simulink subsystem "StreetLaneSegment1x1_asSubsystem"  (R2021a)
settings: Solver=VariableStepAuto  StartTime=0.0  StopTime=10.0  RelTol=1e-3
settings Model: Creator=phill  LastModifiedBy=phill

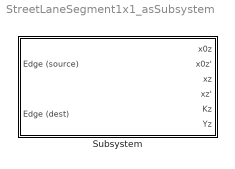
== system StreetLaneSegment1x1_asSubsystem ==
  Subsystem : Subsystem  mask{Kz=10, Tz=5}
      mask prompts: Kz "Kz (Capacity - How many cars fit into this cell)"; Tz "Tz (Nominal travel time for vehicles traveling unobstructed through the cell)"
      mask help:
      | This Block models a single Street-Lane capable of holding / transducing cars (or at least "car volume units") as a cell. This 1x1 version It is connected to a single source edge (over which it can receive cars from a preceeding cell) and a single destination edge (over which it can lose cars to the succeeding cell).  It has a capacity (how many volume-units of cars can be present on the segment at a given time) and a nominal travel time (how long cars would need to travel through it unobstructed). The outputs are:
      |
      | x0z  : how many cars (in car volume units) are "at the end of the cell" (and thus visible for the destination-edge  or the following cell).  The value can only rise if more cars flow in (mind the delay Tz!) than flow out - for instance if a traffic light blocks the exit.
      | x0z' : how many cars flow into (when positive sign) or out of (when negative) the cell
      | xz    : how many cars are in the cell in total (both the ones who just entered and have not reached the end yet, as well as the ones at the end)
      | xz'   : how many cars are flowing into- (positive sign) or out of (negative) the cell per time
      | yz    : the internal flow - how many cars pass into the "endpart" of a cell. It is delayed by Tz compared to the incoming flow y_incoming, so any cars that enter a cell will only "appear visible" at the end of it after that time Tz.
      mask Display:
      | disp('Street Lane Segment 1x1 \n\n');
      | disp(['Kz = ', get_param(gcb,'Kz'), ' | Tz = ', get_param(gcb, 'Tz')])

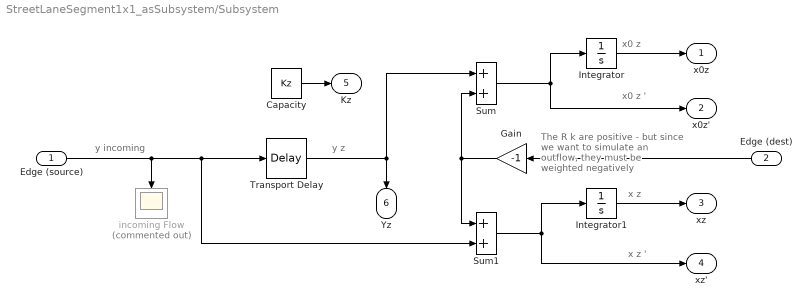
== system StreetLaneSegment1x1_asSubsystem/Subsystem ==
  note: y incoming
  note: x z '
  note: x z
  note: x0 z
  note: x0 z '
  note: y z
  note: The R k are positive - but since we
      | want to simulate an outflow, they
      | must be weighted negatively
  Edge (source) : Inport
  Edge (dest) : Inport  Port=2
  Capacity : Constant  Value=Kz
  Gain : Gain  Gain=-1
  Integrator : Integrator
  Integrator1 : Integrator
  Sum : Sum
  Sum1 : Sum
  Transport Delay : TransportDelay  DelayTime=Tz
  incoming Flow : Scope  Commented=on
  x0z : Outport
  x0z' : Outport  Port=2
  xz : Outport  Port=3
  xz' : Outport  Port=4
  Kz : Outport  Port=5
  Yz : Outport  Port=6
  wires:
  Sum1/1 -> xz'/1, Integrator1/1
  Integrator/1 -> x0z/1
  Transport Delay/1 -> Yz/1, Sum/1
  Edge (dest)/1 -> Gain/1
  Edge (source)/1 -> incoming Flow/1, Sum1/2, Transport Delay/1
  Integrator1/1 -> xz/1
  Gain/1 -> Sum1/1, Sum/2
  Sum/1 -> x0z'/1, Integrator/1
  Capacity/1 -> Kz/1
